simulink model "RL"  (R2025b)
settings: Solver=VariableStepAuto  StartTime=0.0  StopTime=10.0  RelTol=1e-3
model workspace (MAT data in the model file):
  TMax = 500
  theta_max = 45
  thetadot_max = 10
libraries: simulink x3, rllib x1
settings Model: DataDictionary=test.sldd  Creator=rpumpo  LastModifiedBy=rpumpo

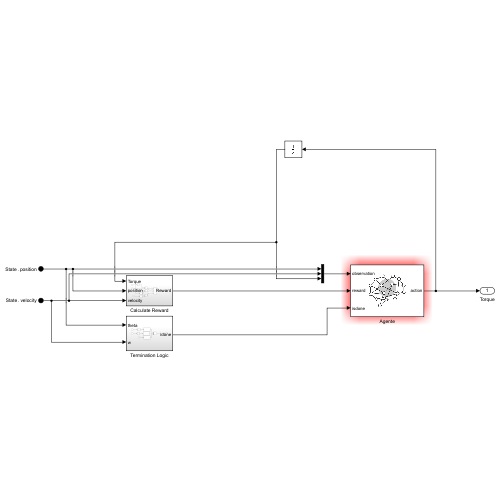
[thumbnail: Simulink's stored preview of the top-level diagram]
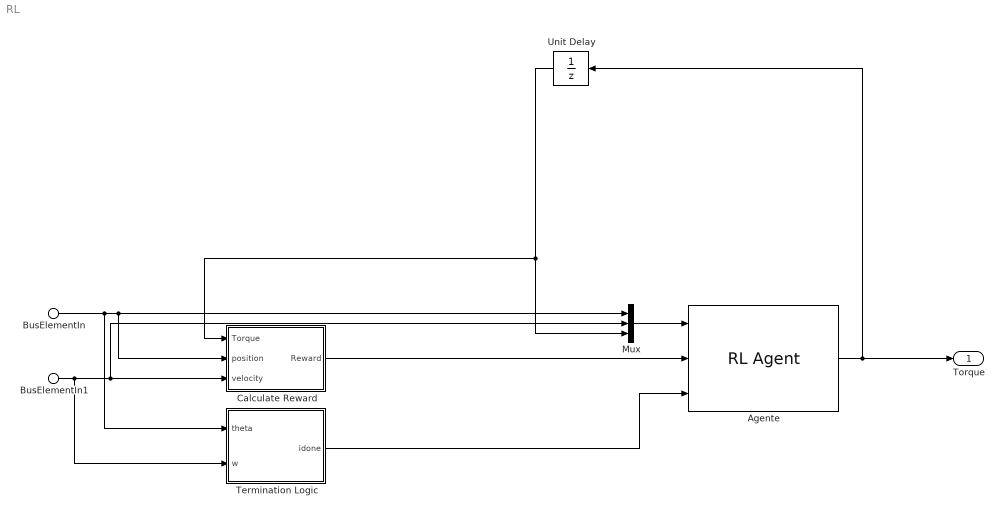
== system RL ==
  BusElementIn : Inport  PortName=State  Element=position
  BusElementIn1 : Inport  PortName=State  Element=velocity
  Agente : rllib/RL Agent  Agent=Agent  ExternalActionAsInput=off  ProvideLastAction=off  ProvideCumRwd=off  TreatAsDirectFeedthrough=on  UseStrictObservationDataTypes=off
  Calculate Reward : Subsystem
  Mux : Mux  Inputs=3
  Termination Logic : Subsystem
  Unit Delay : UnitDelay  SampleTime=-1  HasFrameUpgradeWarning=on
  Torque : Outport  OutDataTypeStr=double
  wires:
  Unit Delay/1 -> Calculate Reward/1(Torque), Mux/3
  Calculate Reward/1(Reward) -> Agente/2
  BusElementIn1/1 -> Mux/2, Calculate Reward/3(velocity), Termination Logic/2(w)
  Termination Logic/1(idone) -> Agente/3
  Agente/1 -> Torque/1, Unit Delay/1
  BusElementIn/1 -> Mux/1, Calculate Reward/2(position), Termination Logic/1(theta)
  Mux/1 -> Agente/1

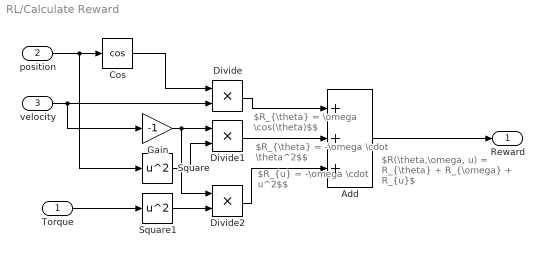
== system RL/Calculate Reward ==
  note: $R_{u} = -\omega \cdot u^2$$
  note: $R_{\theta} = -\omega \cdot \theta^2$$
  note: $R_{\theta} = \omega \cos(\theta)$$
  note: $R(\theta,\omega, u) = R_{\theta} + R_{\omega} + R_{u}$
  Torque : Inport
  position : Inport  Port=2
  velocity : Inport  Port=3
  Add : Sum  Inputs=+++
  Cos : Trigonometry  Operator=cos
  Divide : Product  Inputs=**
  Divide1 : Product  Inputs=**
  Divide2 : Product  Inputs=**
  Gain : Gain  Gain=-1
  Square : Math  Operator=square
  Square1 : Math  Operator=square
  Reward : Outport
  wires:
  Divide1/1 -> Add/2
  Gain/1 -> Divide1/1, Divide2/1
  Add/1 -> Reward/1
  Square/1 -> Divide1/2
  Square1/1 -> Divide2/2
  Divide2/1 -> Add/3
  Divide/1 -> Add/1
  velocity/1 -> Gain/1, Divide/2
  Torque/1 -> Square1/1
  position/1 -> Square/1, Cos/1
  Cos/1 -> Divide/1

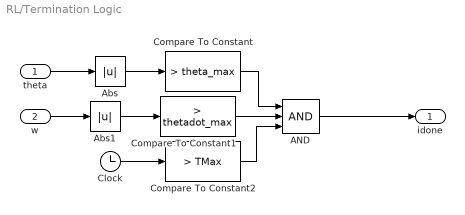
== system RL/Termination Logic ==
  theta : Inport
  w : Inport  Port=2
  AND : Logic  Inputs=3  IconShape=distinctive  AllPortsSameDT=off  OutDataTypeStr=boolean
  Abs : Abs  SaturateOnIntegerOverflow=off
  Abs1 : Abs  SaturateOnIntegerOverflow=off
  Clock : Clock
  Compare To Constant : simulink/Logic and Bit Operations/Compare To Constant  relop=>  const=theta_max  OutDataTypeStr=boolean
  Compare To Constant1 : simulink/Logic and Bit Operations/Compare To Constant  relop=>  const=thetadot_max  OutDataTypeStr=boolean
  Compare To Constant2 : simulink/Logic and Bit Operations/Compare To Constant  relop=>  const=TMax  OutDataTypeStr=boolean
  idone : Outport
  wires:
  theta/1 -> Abs/1
  Abs1/1 -> Compare To Constant1/1
  Clock/1 -> Compare To Constant2/1
  Compare To Constant1/1 -> AND/2
  w/1 -> Abs1/1
  Abs/1 -> Compare To Constant/1
  Compare To Constant/1 -> AND/1
  Compare To Constant2/1 -> AND/3
  AND/1 -> idone/1
